simulink library "SLUGS_Library"  (Simulink 7.8)
settings: Solver=ode45  SolverMode=SingleTasking  StartTime=0.0  StopTime=10.0  RelTol=1e-3
values from neighbouring files (symbols this model uses):
  apSampleTime = 0.01    [mcuInit.m]
  derivativesConstant = 5    [mcuInit.m]
  latlong_WP = 1    [mcuInit.m]
  T = 0.01    [mcuInit.m]
  Xpoints = [0 0]    [mcuInit.m]
  Ypoints = [0 0]    [mcuInit.m]
  Zpoints = [0 0]    [mcuInit.m]
undefined symbols (not defined in the file or in its folder): bankCommandLimit, barAdjust, baroCutTemp, baroOffset, baroScale, barTGain1, barTGain2, barTMean1, barTMean2, baseHeight, baseTemp, daLimit, deLimit, DiscIntNeverNeededParam, drLimit, dtLimit, gaind, getGSLocation, getWP, GS_location, Init_onlyOnce, Init_Reset, IPStar, ISA_g, lapseRate, mass, maxAcc, MaxDwnPthStar, maxDynPressure, maxEta, Ndelay, param, pitAdjust, pitchCommandLimit, pitCutTemp, pitotOffset, pitotScale, pitTGain1, pitTGain2, pitTMean1, pitTMean2, polesd, pressureSensorCutoff, rollControlLimit, SampleT, setDiagnosticFloat, setDiagnosticShort, setLogFloat1, setLogFloat2, setNavLong, setNavNav, tanIntercept, Ts, u1, y1, yawDamperLimit, yo, zerosd
libraries: SLUGS_Library x90, simulink x37, dsPICdrivers x33, aerolibconvert2 x4, aerolibutil x1, aerolibobsolete x1
(part 1 of 7)
settings Model: Creator=Administrator  LastModifiedBy=User

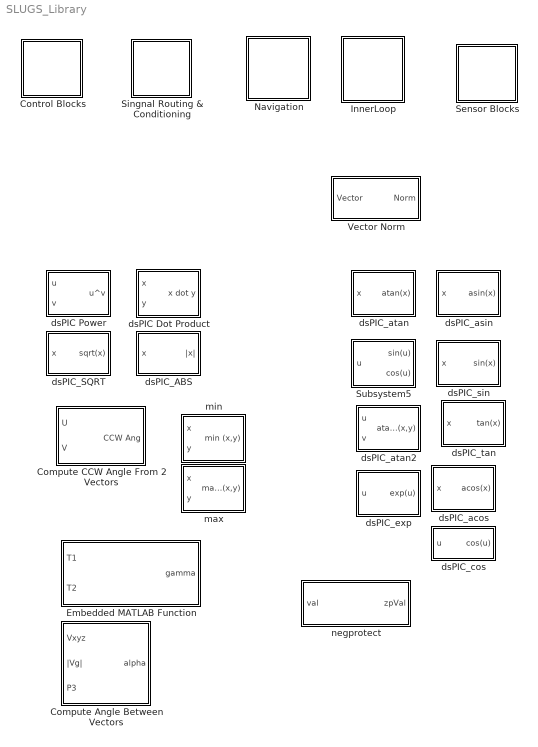
== system SLUGS_Library ==
  Compute Angle Between Vectors : Subsystem
  Compute CCW Angle From 2 Vectors : Subsystem
  Control Blocks : Subsystem
  Embedded MATLAB Function : MATLAB Function  TreatAsAtomicUnit=on
  InnerLoop : Subsystem
  Navigation : Subsystem
  Sensor Blocks : Subsystem  AncestorBlock=SLUGS_Library/Control Blocks
  Singnal Routing & Conditioning : Subsystem
  Subsystem5 : Subsystem
  Vector Norm : Subsystem
  dsPIC Dot Product : Subsystem
  dsPIC Power : Subsystem  AncestorBlock=SLUGS_Library/Air Density from Height/Subsystem
  dsPIC_ABS : Subsystem
  dsPIC_SQRT : Subsystem  AncestorBlock=SLUGS_Library/Compute Airspeed/Subsystem
  dsPIC_acos : Subsystem
  dsPIC_asin : Subsystem  AncestorBlock=SLUGS_Library/Subsystem2
  dsPIC_atan : Subsystem
  dsPIC_atan2 : Subsystem  AncestorBlock=SLUGS_Library/Air Density from Height/Subsystem
  dsPIC_cos : Subsystem  AncestorBlock=SLUGS_Library/Subsystem5
  dsPIC_exp : Subsystem  AncestorBlock=SLUGS_Library/Subsystem11
  dsPIC_sin : Subsystem  AncestorBlock=SLUGS_Library/Subsystem2
  dsPIC_tan : Subsystem
  max : Subsystem  AncestorBlock=SLUGS_Library/Subsystem3
  min : Subsystem  AncestorBlock=SLUGS_Library/Subsystem3
  negprotect : MATLAB Function  TreatAsAtomicUnit=on

== system SLUGS_Library/Compute Angle Between Vectors ==
  Vxyz : Inport
  |Vg| : Inport  Port=2
  P3 : Inport  Port=3
  Product8 : Product  Inputs=*/  RndMeth=Zero
  Product9 : Product  RndMeth=Zero
  Vector Norm : SLUGS_Library/Vector Norm
  "[-1 1]" : Saturate  UpperLimit=1  LowerLimit=-1
  dsPIC Dot Product : SLUGS_Library/dsPIC Dot Product
  dsPIC_acos : SLUGS_Library/dsPIC_acos
  negprotect3 : MATLAB Function  TreatAsAtomicUnit=on
  alpha : Outport
  wires:
  P3/1 -> dsPIC Dot Product/2, Vector Norm/1
  Vxyz/1 -> dsPIC Dot Product/1
  dsPIC Dot Product/1 -> Product8/1
  Vector Norm/1 -> Product9/1
  |Vg|/1 -> Product9/2
  Product9/1 -> negprotect3/1(val)
  Product8/1 -> "[-1 1]"/1
  "[-1 1]"/1 -> dsPIC_acos/1
  negprotect3/1(zpVal) -> Product8/2
  dsPIC_acos/1 -> alpha/1

== system SLUGS_Library/Compute CCW Angle From 2 Vectors ==
  U : Inport
  V : Inport  Port=2
  Add : Sum  Inputs=+-
  Embedded MATLAB Function1 : MATLAB Function  TreatAsAtomicUnit=on
  Selector : Selector  InputPortWidth=3  IndexOptions=Index vector (dialog)  Indices=[1]  OutputSizes=1
  Selector1 : Selector  InputPortWidth=3  IndexOptions=Index vector (dialog)  Indices=[1]  OutputSizes=1
  Selector2 : Selector  InputPortWidth=3  IndexOptions=Index vector (dialog)  Indices=[2]  OutputSizes=1
  Selector3 : Selector  InputPortWidth=3  IndexOptions=Index vector (dialog)  Indices=[2]  OutputSizes=1
  Subsystem1 : SLUGS_Library/Subsystem4
  Subsystem4 : SLUGS_Library/Subsystem4
  CCW Ang : Outport
  wires:
  Embedded MATLAB Function1/1(angle) -> CCW Ang/1
  V/1 -> Selector1/1, Selector2/1
  U/1 -> Selector/1, Selector3/1
  Add/1 -> Embedded MATLAB Function1/1(rawAngle)
  Subsystem1/1 -> Add/2
  Subsystem4/1 -> Add/1
  Selector1/1 -> Subsystem1/2
  Selector2/1 -> Subsystem1/1
  Selector/1 -> Subsystem4/2
  Selector3/1 -> Subsystem4/1

== system SLUGS_Library/Control Blocks ==
  Control Blocks Examples : Subsystem  AncestorBlock=SLUGS_Library/Control Blocks
  Lateral Channel : Subsystem
  Longitudinal Channel : Subsystem
  psi_dot_c Select logic : Subsystem

== system SLUGS_Library/InnerLoop ==
  Lateral Channel : Subsystem  TreatAsAtomicUnit=on
  Longitudinal Channel : Subsystem  TreatAsAtomicUnit=on
  Navigation : Subsystem  TreatAsAtomicUnit=on

== system SLUGS_Library/Navigation ==
  Bank to Psi Dot : Subsystem
  Compute Lateral Error : Subsystem
  Compute Distance : Subsystem  AncestorBlock=SLUGS_Library/Navigation/Compute Distance
  Compute Frenet : Subsystem
  Compute WP Index : Subsystem  AncestorBlock=SLUGS_Library/Navigation/Compute WP Index
  Dot Product : DotProduct  InputSameDT=on  OutDataTypeStr=Inherit: Inherit via internal rule
  Geod2LTP : Subsystem
      mask Description:
      | This block provides transformation of the Geodetic coordinates
      | to the LTP coorinate system. The block uses two consecutive transformations
      | (Geodetic -> ECEF ->LTP).
      | Geodetic coordinates of the LTP origin should also be predetermined.
      mask Help: Oops!
      mask Display: plot(0,0,100,100,[45,40,35,40,40],[85,95,85,95,40],[85,95,85,95,40],[35,40,45,40,40],[60,40,10,20,10,14],[70,40,10,13,10,20],[56,45],[70,70],[60,60],[50,60],[60,60],[30,40],[50,60],[20,20],[30,40],[20,20],[45,55],[35,25],[75,65],[35,25])
  Navigation : Subsystem
  Norm : Subsystem  AncestorBlock=SLUGS_Library/Navigation/Norm
  Normalize Vector : Subsystem
  "Park, Deyst & How Lat Accel Cmd" : Subsystem  AncestorBlock=SLUGS_Library/Navigation/Park, Deyst & How Lat Accel Cmd
  as_c to phi_c : Subsystem
  get WP Coord from Index : Subsystem
  psi_dot to Bank : Subsystem

== system SLUGS_Library/Sensor Blocks ==
  Baro Alt : Subsystem
  Pitot Control End : Subsystem
  Pitot Sensor End : Subsystem

== system SLUGS_Library/Singnal Routing & Conditioning ==
  3D Filter : Subsystem  RTWFcnName=TustinFilter3D  mask{zval=[], pval=-5, kval=5, TSample=0.01}
      mask prompts: zval "Zeros"; pval "Poles"; kval "Gains"; TSample "Sample Time"
      settings: RTWFcnNameOpts=User specified  RTWFileNameOpts=Use function name
      mask Display:
      | droots(zval,pval,kval)
      | port_label('input',1,'3D')
  3D LowPass w/Initial Condition : Subsystem  mask{a=5, yo=yo}
      mask prompts: a "Pole Location (continous)"; yo "Initial condition (3x1)"
      mask help: 3D Discrete 1st Order Low Pass filter
      mask Display:
      | port_label('input',1,'3D')
      | dpoly([a],[1 a],'s')
  Discrete Low Pass w/initial condition : Subsystem  mask{a=0.5, Yo=yo, Ts=T}
      mask prompts: a "Pole location (continuous)"; Yo "Initial condition"; Ts "Sample Time (seconds)"
      mask Display:
      | port_label('input',1,'U')
      | port_label('output',1,'Y')
      | text(0.35,0.85,'Tustin')
      | dpoly([a],[1 a],'s')
  Ellipse Correction : Subsystem  AncestorBlock=SLUGS_Library/Singnal Routing & Conditioning/Ellipse Correction  mask{param=param}
      mask prompts: param "parameter (struct)"
      mask help: Applies the correction from the ellipse algorithm to the raw data being sent through the block. The block expects a 3x1 input vector, and will return a 3x1 output vector. The parameter constant should be a struct with param.xo .yo and .zo being the offsets, param.a .b and .c being the scale factors, and param.phi .rho and .lambda being the angle non-orthogonality (in degrees).
      mask Display:
      | text(0.2,0.85,'Ellipse Correction')
      | port_label('input',1,'RAW')
      | port_label('output',1,'CORR')
  Filter : Subsystem  mask(DiscretizedZeroPole){Zeros=[], Poles=[-5], Gain=5, AbsTol=auto, SampleTime=SampleT, method=tustin, Wc=1}
      mask prompts: Zeros "Zeros (enter in s-main:)"; Poles "Poles (enter in s-domain:)"; Gain "Gain (enter in s-domain:)"; AbsTol "Absolute tolerance:"; SampleTime "Sample time:"; Wc "Critical Frequency (Hz):"
      mask help: Continuous mask uses c2d to transform parameters onto the Discrete Zero-Pole block inside.
      mask init:
      | st=SampleTime;
      | if length(st)>1
      |     st=SampleTime(1);
      | end
      | if(st>0)
      |     [zerosd,polesd,gaind] = sldiscutil('disczpk', {st,method,Wc,Zeros,Poles,Gain});
      | end	
      | s = get_param(gcb,'maskvalues');
      | zeross = s{1};
      | poless = s{2};
      | gainss = s{3};
      | %zerosc = eval(zeross);
      | %polesc = eval(poless);
      | %gainsc = eval(gainss);
      | sldiscutil('initzpkmask', st);
      | if(st==0)
      | set_param([gcb '/Zero Pole'], 'AbsoluteTolerance', AbsTol);
      | end
      mask StyleString: edit,edit,edit,edit,edit,popup(zoh|foh|tustin|prewarp|matched),edit
      mask CallbackString: |||||hidecrit|
      mask Display:
      | droots(zeross,poless,gainss)
      | text( 0.5, 1.0, method, 'verticalAlignment','top')
  Rate Limiter Dynamic with External IC : Subsystem  mask{rlIC=0}
  Saturation : Saturate  SampleTime=SampleT
  Zero Limit : Subsystem
  myMux Fun3 : MATLAB Function  TreatAsAtomicUnit=on

== system SLUGS_Library/Subsystem5 ==
  u : Inport
  C Function Call : dsPICdrivers/OTHERS/C Function Call  Tag=dsPIC_dsPIC_CFunctionCall  FctUpdate=Output Function  fctName='mySin'  INPUT_SIZE=1  INPUT1=real32  INPUT2=--  INPUT3=--  OUTPUT_SIZE=1  OUTPUT1=real32  SampleTime=-1  InputType=[ 7 ]  OutputType=[ 7 ]  FctDeclaration=extern real32_T mySin(real32_T u1);  FctCall=%y1 = mySin(%u1);  OrderingInOutPopup=None  FctStart=None  FctStart_Name=Init_onlyOnce  FctStart_Declaration=inline extern void Init_onlyOnce();  FctStart_Call=Init_onlyOnce();  FctInit=None  FctInit_Name=Init_Reset  FctInit_Declaration=inline extern void Init_Reset();  FctInit_Call=Init_Reset();  PinDigitalInput=[]  PinDigitalOutput=[]  AnalogueInput=[]
  C Function Call1 : dsPICdrivers/OTHERS/C Function Call  Tag=dsPIC_dsPIC_CFunctionCall  FctUpdate=Output Function  fctName='myCos'  INPUT_SIZE=1  INPUT1=real32  INPUT2=--  INPUT3=--  OUTPUT_SIZE=1  OUTPUT1=real32  SampleTime=-1  InputType=[ 7 ]  OutputType=[ 7 ]  FctDeclaration=extern real32_T myCos(real32_T u1);  FctCall=%y1 = myCos(%u1);  OrderingInOutPopup=None  FctStart=None  FctStart_Name=Init_onlyOnce  FctStart_Declaration=inline extern void Init_onlyOnce();  FctStart_Call=Init_onlyOnce();  FctInit=None  FctInit_Name=Init_Reset  FctInit_Declaration=inline extern void Init_Reset();  FctInit_Call=Init_Reset();  PinDigitalInput=[]  PinDigitalOutput=[]  AnalogueInput=[]
  Environment Controller : simulink/Signal Routing/Environment Controller
  Environment Controller1 : simulink/Signal Routing/Environment Controller
  SinCos1 : aerolibobsolete/SinCos
  sin(u) : Outport
  cos(u) : Outport  Port=2
  wires:
  SinCos1/2 -> Environment Controller1/1
  C Function Call1/1 -> Environment Controller1/2
  Environment Controller1/1 -> cos(u)/1
  u/1 -> C Function Call1/1, C Function Call/1, SinCos1/1
  SinCos1/1 -> Environment Controller/1
  C Function Call/1 -> Environment Controller/2
  Environment Controller/1 -> sin(u)/1

== system SLUGS_Library/Vector Norm ==
  Vector : Inport
  dsPIC Dot Product : SLUGS_Library/dsPIC Dot Product
  dsPIC_SQRT : SLUGS_Library/dsPIC_SQRT
  Norm : Outport
  wires:
  dsPIC Dot Product/1 -> dsPIC_SQRT/1
  Vector/1 -> dsPIC Dot Product/1, dsPIC Dot Product/2
  dsPIC_SQRT/1 -> Norm/1

== system SLUGS_Library/dsPIC Dot Product ==
  x : Inport
  y : Inport  Port=2
  Dot Product : DotProduct  InputSameDT=on  OutDataTypeStr=Inherit: Inherit via internal rule
  Embedded MATLAB Function : MATLAB Function  TreatAsAtomicUnit=on
  Environment Controller : simulink/Signal Routing/Environment Controller
  x dot y : Outport
  wires:
  y/1 -> Embedded MATLAB Function/2(y), Dot Product/2
  x/1 -> Embedded MATLAB Function/1(x), Dot Product/1
  Dot Product/1 -> Environment Controller/1
  Embedded MATLAB Function/1(xDoty) -> Environment Controller/2
  Environment Controller/1 -> x dot y/1

== system SLUGS_Library/dsPIC Power ==
  u : Inport
  v : Inport  Port=2
  C Function Call : dsPICdrivers/OTHERS/C Function Call  Tag=dsPIC_dsPIC_CFunctionCall  FctUpdate=Output Function  fctName='myPow'  INPUT_SIZE=1  INPUT1=real32  INPUT2=real32  INPUT3=--  OUTPUT_SIZE=1  OUTPUT1=real32  SampleTime=-1  InputType=[ 7 7 ]  OutputType=[ 7 ]  FctDeclaration=extern real32_T myPow(real32_T u1, real32_T u2);  FctCall=%y1 = myPow(%u1, %u2);  OrderingInOutPopup=None  FctStart=None  FctStart_Name=Init_onlyOnce  FctStart_Declaration=inline extern void Init_onlyOnce();  FctStart_Call=Init_onlyOnce();  FctInit=None  FctInit_Name=Init_Reset  FctInit_Declaration=inline extern void Init_Reset();  FctInit_Call=Init_Reset();  PinDigitalInput=[]  PinDigitalOutput=[]  AnalogueInput=[]
  Environment Controller : simulink/Signal Routing/Environment Controller
  Math Function : Math  Operator=pow  SaturateOnIntegerOverflow=on
  u^v : Outport
  wires:
  u/1 -> C Function Call/1, Math Function/1
  v/1 -> C Function Call/2, Math Function/2
  Math Function/1 -> Environment Controller/1
  C Function Call/1 -> Environment Controller/2
  Environment Controller/1 -> u^v/1

== system SLUGS_Library/dsPIC_ABS ==
  x : Inport
  Abs : Abs
  C Function Call : dsPICdrivers/OTHERS/C Function Call  Tag=dsPIC_dsPIC_CFunctionCall  FctUpdate=Output Function  fctName='myAbs'  INPUT_SIZE=1  INPUT1=real32  INPUT2=--  INPUT3=--  OUTPUT_SIZE=1  OUTPUT1=real32  SampleTime=-1  InputType=[ 7 ]  OutputType=[ 7 ]  FctDeclaration=extern real32_T myAbs(real32_T u1);  FctCall=%y1 = myAbs(%u1);  OrderingInOutPopup=None  FctStart=None  FctStart_Name=Init_onlyOnce  FctStart_Declaration=inline extern void Init_onlyOnce();  FctStart_Call=Init_onlyOnce();  FctInit=None  FctInit_Name=Init_Reset  FctInit_Declaration=inline extern void Init_Reset();  FctInit_Call=Init_Reset();  PinDigitalInput=[]  PinDigitalOutput=[]  AnalogueInput=[]
  Environment Controller : simulink/Signal Routing/Environment Controller
  |x| : Outport
  wires:
  x/1 -> Abs/1, C Function Call/1
  C Function Call/1 -> Environment Controller/2
  Abs/1 -> Environment Controller/1
  Environment Controller/1 -> |x|/1

== system SLUGS_Library/dsPIC_SQRT ==
  x : Inport
  C Function Call : dsPICdrivers/OTHERS/C Function Call  Tag=dsPIC_dsPIC_CFunctionCall  FctUpdate=Output Function  fctName='mySqrt'  INPUT_SIZE=1  INPUT1=real32  INPUT2=--  INPUT3=--  OUTPUT_SIZE=1  OUTPUT1=real32  SampleTime=-1  InputType=[ 7 ]  OutputType=[ 7 ]  FctDeclaration=extern real32_T mySqrt(real32_T u1);  FctCall=%y1 = mySqrt(%u1);  OrderingInOutPopup=None  FctStart=None  FctStart_Name=Init_onlyOnce  FctStart_Declaration=inline extern void Init_onlyOnce();  FctStart_Call=Init_onlyOnce();  FctInit=None  FctInit_Name=Init_Reset  FctInit_Declaration=inline extern void Init_Reset();  FctInit_Call=Init_Reset();  PinDigitalInput=[]  PinDigitalOutput=[]  AnalogueInput=[]
  Environment Controller : simulink/Signal Routing/Environment Controller
  Math Function1 : Math  Operator=sqrt  SaturateOnIntegerOverflow=on
  negprotect : MATLAB Function  TreatAsAtomicUnit=on
  sqrt(x) : Outport
  wires:
  C Function Call/1 -> Environment Controller/2
  Math Function1/1 -> Environment Controller/1
  Environment Controller/1 -> sqrt(x)/1
  negprotect/1(zpVal) -> C Function Call/1, Math Function1/1
  x/1 -> negprotect/1(val)

== system SLUGS_Library/dsPIC_acos ==
  x : Inport
  C Function Call : dsPICdrivers/OTHERS/C Function Call  Tag=dsPIC_dsPIC_CFunctionCall  FctUpdate=Output Function  fctName='myAcos'  INPUT_SIZE=1  INPUT1=real32  INPUT2=--  INPUT3=--  OUTPUT_SIZE=1  OUTPUT1=real32  SampleTime=-1  InputType=[ 7 ]  OutputType=[ 7 ]  FctDeclaration=extern real32_T myAcos(real32_T u1);  FctCall=%y1 = myAcos(%u1);  OrderingInOutPopup=None  FctStart=None  FctStart_Name=Init_onlyOnce  FctStart_Declaration=inline extern void Init_onlyOnce();  FctStart_Call=Init_onlyOnce();  FctInit=None  FctInit_Name=Init_Reset  FctInit_Declaration=inline extern void Init_Reset();  FctInit_Call=Init_Reset();  PinDigitalInput=[]  PinDigitalOutput=[]  AnalogueInput=[]
  Environment Controller : simulink/Signal Routing/Environment Controller
  Trigonometric Function : Trigonometry  Operator=acos
  acos(x) : Outport
  wires:
  x/1 -> C Function Call/1, Trigonometric Function/1
  Trigonometric Function/1 -> Environment Controller/1
  C Function Call/1 -> Environment Controller/2
  Environment Controller/1 -> acos(x)/1

== system SLUGS_Library/dsPIC_asin ==
  x : Inport
  C Function Call : dsPICdrivers/OTHERS/C Function Call  Tag=dsPIC_dsPIC_CFunctionCall  FctUpdate=Output Function  fctName='myAsin'  INPUT_SIZE=1  INPUT1=real32  INPUT2=--  INPUT3=--  OUTPUT_SIZE=1  OUTPUT1=real32  SampleTime=-1  InputType=[ 7 ]  OutputType=[ 7 ]  FctDeclaration=extern real32_T myAsin(real32_T u1);  FctCall=%y1 = myAsin(%u1);  OrderingInOutPopup=None  FctStart=None  FctStart_Name=Init_onlyOnce  FctStart_Declaration=inline extern void Init_onlyOnce();  FctStart_Call=Init_onlyOnce();  FctInit=None  FctInit_Name=Init_Reset  FctInit_Declaration=inline extern void Init_Reset();  FctInit_Call=Init_Reset();  PinDigitalInput=[]  PinDigitalOutput=[]  AnalogueInput=[]
  Environment Controller : simulink/Signal Routing/Environment Controller
  Trigonometric Function : Trigonometry  Operator=asin
  "[-1,1]" : Saturate  UpperLimit=0.9999  LowerLimit=-0.999
  asin(x) : Outport
  wires:
  Environment Controller/1 -> asin(x)/1
  C Function Call/1 -> Environment Controller/2
  Trigonometric Function/1 -> Environment Controller/1
  x/1 -> "[-1,1]"/1
  "[-1,1]"/1 -> Trigonometric Function/1, C Function Call/1

== system SLUGS_Library/dsPIC_atan ==
  x : Inport
  C Function Call : dsPICdrivers/OTHERS/C Function Call  Tag=dsPIC_dsPIC_CFunctionCall  FctUpdate=Output Function  fctName='myAtan'  INPUT_SIZE=1  INPUT1=real32  INPUT2=--  INPUT3=--  OUTPUT_SIZE=1  OUTPUT1=real32  SampleTime=-1  InputType=[ 7 ]  OutputType=[ 7 ]  FctDeclaration=extern real32_T myAtan(real32_T u1);  FctCall=%y1 = myAtan(%u1);  OrderingInOutPopup=None  FctStart=None  FctStart_Name=Init_onlyOnce  FctStart_Declaration=inline extern void Init_onlyOnce();  FctStart_Call=Init_onlyOnce();  FctInit=None  FctInit_Name=Init_Reset  FctInit_Declaration=inline extern void Init_Reset();  FctInit_Call=Init_Reset();  PinDigitalInput=[]  PinDigitalOutput=[]  AnalogueInput=[]
  Environment Controller : simulink/Signal Routing/Environment Controller
  Trigonometric Function : Trigonometry  Operator=atan
  atan(x) : Outport
  wires:
  Environment Controller/1 -> atan(x)/1
  C Function Call/1 -> Environment Controller/2
  Trigonometric Function/1 -> Environment Controller/1
  x/1 -> Trigonometric Function/1, C Function Call/1

== system SLUGS_Library/dsPIC_atan2 ==
  u : Inport
  v : Inport  Port=2
  C Function Call : dsPICdrivers/OTHERS/C Function Call  Tag=dsPIC_dsPIC_CFunctionCall  FctUpdate=Output Function  fctName='myAtan2'  INPUT_SIZE=1  INPUT1=real32  INPUT2=real32  INPUT3=--  OUTPUT_SIZE=1  OUTPUT1=real32  SampleTime=-1  InputType=[ 7 7 ]  OutputType=[ 7 ]  FctDeclaration=extern real32_T myAtan2(real32_T u1, real32_T u2);  FctCall=%y1 = myAtan2(%u1, %u2);  OrderingInOutPopup=None  FctStart=None  FctStart_Name=Init_onlyOnce  FctStart_Declaration=inline extern void Init_onlyOnce();  FctStart_Call=Init_onlyOnce();  FctInit=None  FctInit_Name=Init_Reset  FctInit_Declaration=inline extern void Init_Reset();  FctInit_Call=Init_Reset();  PinDigitalInput=[]  PinDigitalOutput=[]  AnalogueInput=[]
  Environment Controller : simulink/Signal Routing/Environment Controller
  Trigonometric Function : Trigonometry  Operator=atan2
  atan2(x,y) : Outport
  wires:
  u/1 -> Trigonometric Function/1, C Function Call/1
  v/1 -> Trigonometric Function/2, C Function Call/2
  Trigonometric Function/1 -> Environment Controller/1
  C Function Call/1 -> Environment Controller/2
  Environment Controller/1 -> atan2(x,y)/1

== system SLUGS_Library/dsPIC_cos ==
  u : Inport
  Environment Controller1 : simulink/Signal Routing/Environment Controller
  Trigonometric Function : Trigonometry  Operator=cos
  "[apUtils.c]" : dsPICdrivers/OTHERS/C Function Call  Tag=dsPIC_dsPIC_CFunctionCall  FctUpdate=Output Function  fctName='myCos'  INPUT_SIZE=1  INPUT1=real32  INPUT2=--  INPUT3=--  OUTPUT_SIZE=1  OUTPUT1=real32  SampleTime=-1  InputType=[ 7 ]  OutputType=[ 7 ]  FctDeclaration=extern real32_T myCos(real32_T u1);  FctCall=%y1 = myCos(%u1);  OrderingInOutPopup=None  FctStart=None  FctStart_Name=Init_onlyOnce  FctStart_Declaration=inline extern void Init_onlyOnce();  FctStart_Call=Init_onlyOnce();  FctInit=None  FctInit_Name=Init_Reset  FctInit_Declaration=inline extern void Init_Reset();  FctInit_Call=Init_Reset();  PinDigitalInput=[]  PinDigitalOutput=[]  AnalogueInput=[]
  cos(u) : Outport
  wires:
  Trigonometric Function/1 -> Environment Controller1/1
  "[apUtils.c]"/1 -> Environment Controller1/2
  Environment Controller1/1 -> cos(u)/1
  u/1 -> Trigonometric Function/1, "[apUtils.c]"/1

== system SLUGS_Library/dsPIC_exp ==
  u : Inport
  C Function Call : dsPICdrivers/OTHERS/C Function Call  Tag=dsPIC_dsPIC_CFunctionCall  FctUpdate=Output Function  fctName='myExp'  INPUT_SIZE=1  INPUT1=real32  INPUT2=--  INPUT3=--  OUTPUT_SIZE=1  OUTPUT1=real32  SampleTime=-1  InputType=[ 7 ]  OutputType=[ 7 ]  FctDeclaration=extern real32_T myExp(real32_T u1);  FctCall=%y1 = myExp(%u1);  OrderingInOutPopup=None  FctStart=None  FctStart_Name=Init_onlyOnce  FctStart_Declaration=inline extern void Init_onlyOnce();  FctStart_Call=Init_onlyOnce();  FctInit=None  FctInit_Name=Init_Reset  FctInit_Declaration=inline extern void Init_Reset();  FctInit_Call=Init_Reset();  PinDigitalInput=[]  PinDigitalOutput=[]  AnalogueInput=[]
  Environment Controller : simulink/Signal Routing/Environment Controller
  Math Function : Math  SaturateOnIntegerOverflow=on
  exp(u) : Outport
  wires:
  C Function Call/1 -> Environment Controller/2
  Environment Controller/1 -> exp(u)/1
  u/1 -> C Function Call/1, Math Function/1
  Math Function/1 -> Environment Controller/1

== system SLUGS_Library/dsPIC_sin ==
  x : Inport
  C Function Call : dsPICdrivers/OTHERS/C Function Call  Tag=dsPIC_dsPIC_CFunctionCall  FctUpdate=Output Function  fctName='mySin'  INPUT_SIZE=1  INPUT1=real32  INPUT2=--  INPUT3=--  OUTPUT_SIZE=1  OUTPUT1=real32  SampleTime=-1  InputType=[ 7 ]  OutputType=[ 7 ]  FctDeclaration=extern real32_T mySin(real32_T u1);  FctCall=%y1 = mySin(%u1);  OrderingInOutPopup=None  FctStart=None  FctStart_Name=Init_onlyOnce  FctStart_Declaration=inline extern void Init_onlyOnce();  FctStart_Call=Init_onlyOnce();  FctInit=None  FctInit_Name=Init_Reset  FctInit_Declaration=inline extern void Init_Reset();  FctInit_Call=Init_Reset();  PinDigitalInput=[]  PinDigitalOutput=[]  AnalogueInput=[]
  Environment Controller : simulink/Signal Routing/Environment Controller
  Trigonometric Function : Trigonometry
  sin(x) : Outport
  wires:
  Environment Controller/1 -> sin(x)/1
  C Function Call/1 -> Environment Controller/2
  Trigonometric Function/1 -> Environment Controller/1
  x/1 -> Trigonometric Function/1, C Function Call/1

== system SLUGS_Library/dsPIC_tan ==
  x : Inport
  C Function Call : dsPICdrivers/OTHERS/C Function Call  Tag=dsPIC_dsPIC_CFunctionCall  FctUpdate=Output Function  fctName='myTan'  INPUT_SIZE=1  INPUT1=real32  INPUT2=--  INPUT3=--  OUTPUT_SIZE=1  OUTPUT1=real32  SampleTime=-1  InputType=[ 7 ]  OutputType=[ 7 ]  FctDeclaration=extern real32_T myTan(real32_T u1);  FctCall=%y1 = myTan(%u1);  OrderingInOutPopup=None  FctStart=None  FctStart_Name=Init_onlyOnce  FctStart_Declaration=inline extern void Init_onlyOnce();  FctStart_Call=Init_onlyOnce();  FctInit=None  FctInit_Name=Init_Reset  FctInit_Declaration=inline extern void Init_Reset();  FctInit_Call=Init_Reset();  PinDigitalInput=[]  PinDigitalOutput=[]  AnalogueInput=[]
  Environment Controller : simulink/Signal Routing/Environment Controller
  Trigonometric Function : Trigonometry  Operator=tan
  tan(x) : Outport
  wires:
  x/1 -> C Function Call/1, Trigonometric Function/1
  Trigonometric Function/1 -> Environment Controller/1
  C Function Call/1 -> Environment Controller/2
  Environment Controller/1 -> tan(x)/1

== system SLUGS_Library/max ==
  x : Inport
  y : Inport  Port=2
  Relational Operator : RelationalOperator  Operator=>  OutDataTypeStr=boolean
  Switch : Switch  Threshold=0.5
  max (x,y) : Outport
  wires:
  x/1 -> Relational Operator/1, Switch/1
  y/1 -> Relational Operator/2, Switch/3
  Relational Operator/1 -> Switch/2
  Switch/1 -> max (x,y)/1

== system SLUGS_Library/min ==
  x : Inport
  y : Inport  Port=2
  Relational Operator : RelationalOperator  Operator=<  OutDataTypeStr=boolean
  Switch : Switch  Threshold=0.5
  min (x,y) : Outport
  wires:
  Switch/1 -> min (x,y)/1
  Relational Operator/1 -> Switch/2
  y/1 -> Switch/3, Relational Operator/2
  x/1 -> Switch/1, Relational Operator/1

== system SLUGS_Library/Control Blocks/Control Blocks Examples ==
  PD Controller  Internal Derivative : Subsystem  mask{TSample=SampleT, NDelay=5}
      mask prompts: TSample "Sample Time"; NDelay "Derivation Time Constant Factor (1->10)"
      mask help:
      | This Block implements a PD Controller with the Following Characteristcs:
      |
      | 1.- It still expects 3 values for Gains. The second term (I) is ignored
      | 2.- The time Derivative is "low-passed" by using the previous N samples instead of the one before
  PD Controller  no Internal Derivative : Subsystem  mask{TSample=SampleT}
      mask prompts: TSample "Sample Time"
      mask help:
      | This Block implements a PD Controller with the Following Characteristcs:
      |
      | 1.- It still expects 3 values for Gains. The second term (I) is ignored
      | 2.- The time Derivative is "low-passed" by using the previous N samples instead of the one before
  PI Controller : Subsystem  mask{TSample=SampleT, upperLimit=10, lowerLimit=-10}
      mask prompts: TSample "Sample Time"; upperLimit "Integrator Upper Windup Limit"; lowerLimit "Integrator Lower Windup Limit"
      mask help:
      | This Block implements a PI Controller with the Following Characteristcs:
      |
      | 1.- Integrator antiwindup is given by the limits in the block
      | 2.-The gain still expects 3 values (the D term is ignored)
      | 3.- It contains an Integrator Reset if needed
  PI Controller w/Anti-Windup : Subsystem  mask(PID){Tsample=Ts, Ndelay=Ndelay, upperSaturationLimit=deLimit, lowerSaturationLimit=0}
      mask prompts: Tsample "Sample Time"; Ndelay "Integer delays for de/dt"; upperSaturationLimit "Upper Saturation Limit"; lowerSaturationLimit "Lower Saturation Limit"
      mask help: PID controller block with anti-windup and saturation limits. Implemented as a discrete forwardl integration which stops integrating when the output is saturated. Derivative is implemented as a numerical derivative with N integer delays to smooth output.
      mask Display:
      | disp('PI')
      | port_label('input',1,'error')
      | port_label('input',3,'gains')
      | port_label('input',2,'reset')
      | port_label('input',4,'trim')
      | port_label('output',1,'output')
  PID Controller : Subsystem  mask{TSample=SampleT, NDelay=5, upperLimit=10, lowerLimit=-10}
      mask prompts: TSample "Sample Time"; NDelay "Derivation Time Constant Factor (1->10)"; upperLimit "Integrator Upper Windup Limit"; lowerLimit "Integrator Lower Windup Limit"
      mask help:
      | This Block implements a PID Controller with the Following Characteristcs:
      |
      | 1.- Integrator antiwindup is given by the limits in the block
      | 2.- The time Derivative is "low-passed" by using the previous N samples instead of the one before
      | 3.- It contains an Integrator Reset if needed
  PID Controller no Internal Derivative : Subsystem  mask{TSample=SampleT, upperLimit=10, lowerLimit=-10}
      mask prompts: TSample "Sample Time"; upperLimit "Integrator Upper Windup Limit"; lowerLimit "Integrator Lower Windup Limit"
      mask help:
      | This Block implements a PID Controller with the Following Characteristcs:
      |
      | 1.- Integrator antiwindup is given by the limits in the block
      | 2.- The error time derivative is provided and therefore no derivtive block is implemented
      | 3.- It contains an Integrator Reset if needed
  PID Controller w/Anti-Windup : Subsystem  mask(PID){Tsample=Ts, Ndelay=Ndelay, upperSaturationLimit=deLimit, lowerSaturationLimit=0}
      mask prompts: Tsample "Sample Time"; Ndelay "Integer delays for de/dt"; upperSaturationLimit "Upper Saturation Limit"; lowerSaturationLimit "Lower Saturation Limit"
      mask help: PID controller block with anti-windup and saturation limits. Implemented as a discrete forwardl integration which stops integrating when the output is saturated. Derivative is implemented as a numerical derivative with N integer delays to smooth output.
      mask Display:
      | disp('PID')
      | port_label('input',1,'error')
      | port_label('input',3,'gains')
      | port_label('input',2,'reset')
      | port_label('input',4,'trim')
      | port_label('output',1,'output')
  PID available Derivative w/Anti-Windup : Subsystem  mask(PID){Tsample=Ts, Ndelay=Ndelay, SaturationLimit=deLimit}
      mask prompts: Tsample "Sample Time"; Ndelay "Integer delays for de/dt"; SaturationLimit "Saturation Limit"
      mask help: PID controller block with anti-windup and saturation limits. Implemented as a discrete forwardl integration which stops integrating when the output is saturated. Derivative is implemented as a numerical derivative with N integer delays to smooth output.
      mask Display:
      | disp('PID')
      | port_label('input',1,'error')
      | port_label('input',2,'de/dt')
      | port_label('input',3,'gains')
      | port_label('input',4,'reset')
      | port_label('output',1,'output')

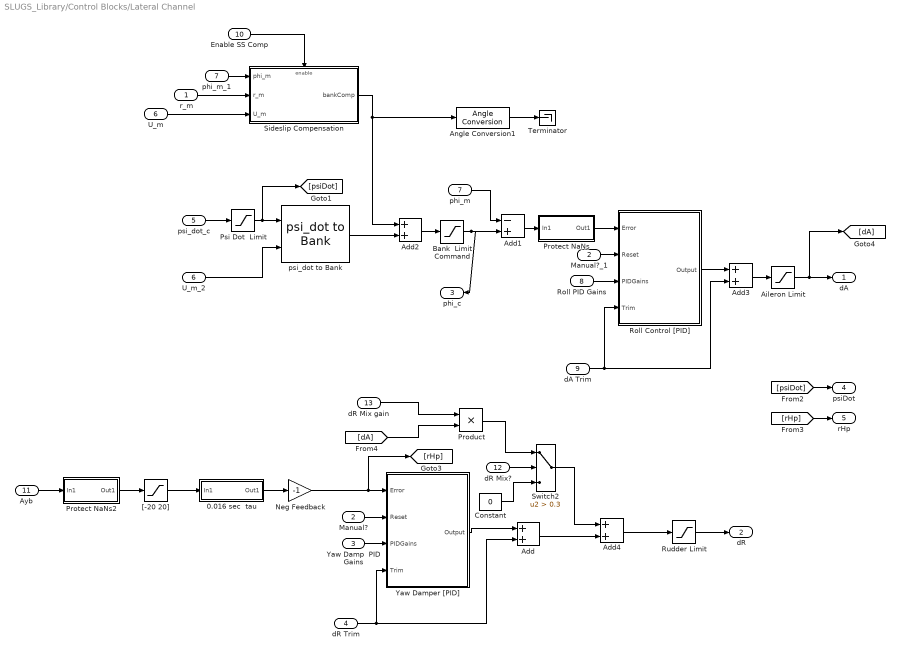
== system SLUGS_Library/Control Blocks/Lateral Channel ==
  r_m : Inport
  Manual? : Inport  Port=2
  Yaw Damp  PID Gains : Inport  Port=3
  dR Trim : Inport  Port=4
  psi_dot_c : Inport  Port=5
  U_m : Inport  Port=6
  phi_m : Inport  Port=7
  Roll PID Gains : Inport  Port=8
  dA Trim : Inport  Port=9
  Enable SS Comp : Inport  Port=10
  Ayb : Inport  Port=11
  dR Mix? : Inport  Port=12
  dR Mix gain : Inport  Port=13
  0.016 sec  tau : Subsystem  mask(Tustin1stOrderLowpassAutoInitialCondition){f=10, T=T}
      mask prompts: f "Lowpass Frequency"; T "Sample Time"
      mask help: Takes a 3db rolloff frequency (in Hz, NOT radians/s) and a sample time. Performs a symbolic Tustin conversion and implements in a discrete filter. The initial output of the filter is set by the first sample.
      mask Help: Enter the desired 3db rolloff frequency in Hz and the sample time. Initial conditions are sampled automatically.
      mask Display: fprintf('%.2f Hz lowpass',f)
  Add{,2..4} (4 alike) : Sum  OutDataTypeStr=single
  Add1 : Sum  Inputs=-+  OutDataTypeStr=single
  Aileron Limit : Saturate  UpperLimit=daLimit  LowerLimit=-daLimit  SampleTime=apSampleTime
  Angle Conversion1 : aerolibconvert2/Angle Conversion  IU=rad  OU=deg
  Bank  Limit Command : Saturate  UpperLimit=bankCommandLimit  LowerLimit=-bankCommandLimit  SampleTime=apSampleTime
  Constant : Constant  Value=0  OutDataTypeStr=single
  Manual?_1 : InportShadow  Port=2
  "Neg Feedback " : Gain  Gain=-1  OutDataTypeStr=float('single')
  Product : Product  RndMeth=Zero
  Protect NaNs : Subsystem
  Protect NaNs2 : Subsystem
  Psi Dot  Limit : Saturate  UpperLimit=1  LowerLimit=-1  SampleTime=apSampleTime
  Roll Control [PID] : Subsystem  AncestorBlock=SLUGS_Library/Control Blocks/PID Controller w//Anti-Windup  mask(PID){Tsample=apSampleTime, Ndelay=derivativesConstant, upperSaturationLimit=daLimit, lowerSaturationLimit=-daLimit}
      mask prompts: Tsample "Sample Time"; Ndelay "Integer delays for de/dt"; upperSaturationLimit "Upper Saturation Limit"; lowerSaturationLimit "Lower Saturation Limit"
      mask help: PID controller block with anti-windup and saturation limits. Implemented as a discrete forwardl integration which stops integrating when the output is saturated. Derivative is implemented as a numerical derivative with N integer delays to smooth output.
      mask Display:
      | disp('PID')
      | port_label('input',1,'error')
      | port_label('input',3,'gains')
      | port_label('input',2,'reset')
      | port_label('input',4,'trim')
      | port_label('output',1,'output')
  Rudder Limit : Saturate  UpperLimit=drLimit  LowerLimit=-drLimit  SampleTime=apSampleTime
  Sideslip Compensation : Subsystem
  Switch2 : Switch  Criteria=u2 > Threshold  Threshold=0.3  InputSameDT=on
  Terminator : Terminator
  U_m_2 : InportShadow  Port=6
  Yaw Damper [PID] : Subsystem  AncestorBlock=SLUGS_Library/Control Blocks/PID Controller w//Anti-Windup  mask(PID){Tsample=apSampleTime, Ndelay=derivativesConstant, upperSaturationLimit=drLimit, lowerSaturationLimit=-drLimit}
      mask prompts: Tsample "Sample Time"; Ndelay "Integer delays for de/dt"; upperSaturationLimit "Upper Saturation Limit"; lowerSaturationLimit "Lower Saturation Limit"
      mask help: PID controller block with anti-windup and saturation limits. Implemented as a discrete forwardl integration which stops integrating when the output is saturated. Derivative is implemented as a numerical derivative with N integer delays to smooth output.
      mask Display:
      | disp('PID')
      | port_label('input',1,'error')
      | port_label('input',3,'gains')
      | port_label('input',2,'reset')
      | port_label('input',4,'trim')
      | port_label('output',1,'output')
  "[-20 20]" : Saturate  UpperLimit=20  LowerLimit=-20
  phi_m_1 : InportShadow  Port=7
  psi_dot to Bank : SLUGS_Library/Navigation/psi_dot to Bank
  dA : Outport
  dR : Outport  Port=2
  phi_c : Outport  Port=3
  psiDot : Outport  Port=4
  rHp : Outport  Port=5
  wires:
  psi_dot_c/1 -> Psi Dot  Limit/1
  Psi Dot  Limit/1 -> psi_dot to Bank/1, [psiDot]
  Bank  Limit Command/1 -> Add1/2, phi_c/1
  phi_m/1 -> Add1/1
  Add1/1 -> Protect NaNs/1(In1)
  Aileron Limit/1 -> dA/1, [dA]
  dA Trim/1 -> Add3/2, Roll Control [PID]/4(Trim)
  Roll Control [PID]/1(Output) -> Add3/1
  Add3/1 -> Aileron Limit/1
  Roll PID Gains/1 -> Roll Control [PID]/3(PIDGains)
  Manual?_1/1 -> Roll Control [PID]/2(Reset)
  dR Trim/1 -> Add/2, Yaw Damper [PID]/4(Trim)
  Yaw Damper [PID]/1(Output) -> Add/1
  Yaw Damp  PID Gains/1 -> Yaw Damper [PID]/3(PIDGains)
  Manual?/1 -> Yaw Damper [PID]/2(Reset)
  U_m_2/1 -> psi_dot to Bank/2
  Add2/1 -> Bank  Limit Command/1
  psi_dot to Bank/1 -> Add2/2
  Sideslip Compensation/1(bankComp) -> Add2/1, Angle Conversion1/1
  phi_m_1/1 -> Sideslip Compensation/1(phi_m)
  r_m/1 -> Sideslip Compensation/2(r_m)
  U_m/1 -> Sideslip Compensation/3(U_m)
  Enable SS Comp/1 -> Sideslip Compensation/Enable
  Ayb/1 -> Protect NaNs2/1(In1)
  "Neg Feedback "/1 -> [rHp], Yaw Damper [PID]/1(Error)
  0.016 sec  tau/1(Out1) -> "Neg Feedback "/1
  Rudder Limit/1 -> dR/1
  Protect NaNs/1(Out1) -> Roll Control [PID]/1(Error)
  Protect NaNs2/1(Out1) -> "[-20 20]"/1
  "[-20 20]"/1 -> 0.016 sec  tau/1(In1)
  Angle Conversion1/1 -> Terminator/1
  Add4/1 -> Rudder Limit/1
  Add/1 -> Add4/2
  Switch2/1 -> Add4/1
  dR Mix?/1 -> Switch2/2
  Constant/1 -> Switch2/3
  Product/1 -> Switch2/1
  dR Mix gain/1 -> Product/1
  [dA] -> Product/2
  [psiDot] -> psiDot/1
  [rHp] -> rHp/1

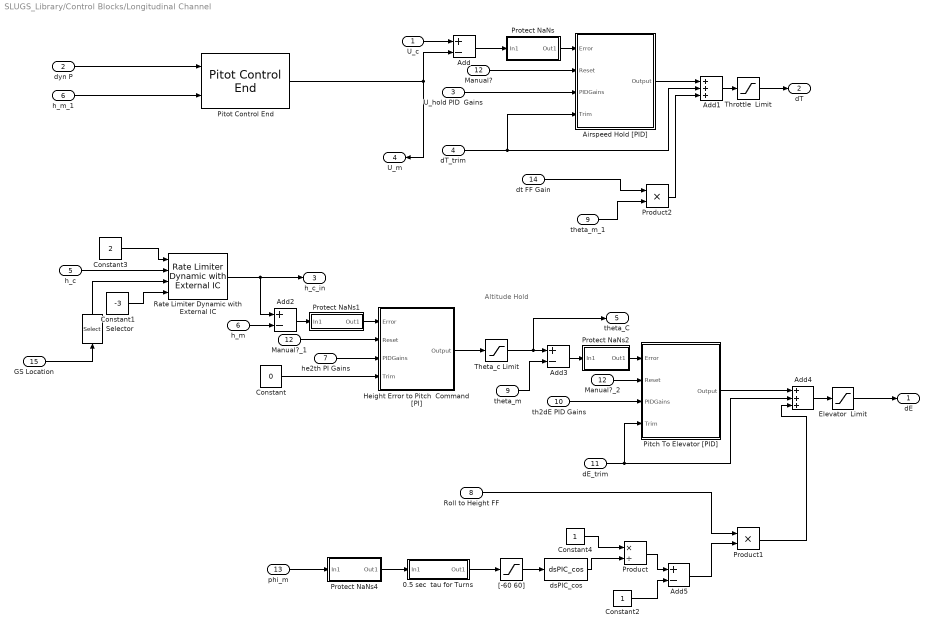
== system SLUGS_Library/Control Blocks/Longitudinal Channel ==
  note: Altitude Hold
  U_c : Inport
  dyn P : Inport  Port=2
  U_hold PID  Gains : Inport  Port=3
  dT_trim : Inport  Port=4
  h_c : Inport  Port=5
  h_m : Inport  Port=6
  he2th PI Gains : Inport  Port=7
  Roll to Height FF : Inport  Port=8
  theta_m : Inport  Port=9
  th2dE PID Gains : Inport  Port=10
  dE_trim : Inport  Port=11
  Manual? : Inport  Port=12
  phi_m : Inport  Port=13
  dt FF Gain : Inport  Port=14
  GS Location : Inport  Port=15
  0.5 sec  tau for Turns : Subsystem  mask(Tustin1stOrderLowpassAutoInitialCondition){f=0.32, T=T}
      mask prompts: f "Lowpass Frequency"; T "Sample Time"
      mask help: Takes a 3db rolloff frequency (in Hz, NOT radians/s) and a sample time. Performs a symbolic Tustin conversion and implements in a discrete filter. The initial output of the filter is set by the first sample.
      mask Help: Enter the desired 3db rolloff frequency in Hz and the sample time. Initial conditions are sampled automatically.
      mask Display: fprintf('%.2f Hz lowpass',f)
  Add : Sum  Inputs=+-
  Add1 : Sum  Inputs=3  OutDataTypeStr=single
  Add2 : Sum  Inputs=+-  OutDataTypeStr=single
  Add3 : Sum  Inputs=+-  OutDataTypeStr=single
  Add4 : Sum  Inputs=3  OutDataTypeStr=single
  Add5 : Sum  Inputs=+-  OutDataTypeStr=single
  Airspeed Hold [PID] : Subsystem  AncestorBlock=SLUGS_Library/Control Blocks/PID Controller w//Anti-Windup  mask(PID){Tsample=apSampleTime, Ndelay=derivativesConstant, upperSaturationLimit=dtLimit, lowerSaturationLimit=0}
      mask prompts: Tsample "Sample Time"; Ndelay "Integer delays for de/dt"; upperSaturationLimit "Upper Saturation Limit"; lowerSaturationLimit "Lower Saturation Limit"
      mask help: PID controller block with anti-windup and saturation limits. Implemented as a discrete forwardl integration which stops integrating when the output is saturated. Derivative is implemented as a numerical derivative with N integer delays to smooth output.
      mask Display:
      | disp('PID')
      | port_label('input',1,'error')
      | port_label('input',3,'gains')
      | port_label('input',2,'reset')
      | port_label('input',4,'trim')
      | port_label('output',1,'output')
  Constant : Constant  Value=0
  Constant1 : Constant  Value=-3  OutDataTypeStr=single
  Constant2 : Constant  OutDataTypeStr=single
  Constant3 : Constant  Value=2  OutDataTypeStr=single
  Constant4 : Constant  OutDataTypeStr=single
  Elevator  Limit : Saturate  UpperLimit=deLimit  LowerLimit=-deLimit  SampleTime=apSampleTime
  Height Error to Pitch  Command [PI] : Subsystem  AncestorBlock=SLUGS_Library/Control Blocks/PI Controller w//Anti-Windup  mask(PID){Tsample=apSampleTime, Ndelay=derivativesConstant, upperSaturationLimit=pitchCommandLimit, lowerSaturationLimit=-pitchCommandLimit}
      mask prompts: Tsample "Sample Time"; Ndelay "Integer delays for de/dt"; upperSaturationLimit "Upper Saturation Limit"; lowerSaturationLimit "Lower Saturation Limit"
      mask help: PID controller block with anti-windup and saturation limits. Implemented as a discrete forwardl integration which stops integrating when the output is saturated. Derivative is implemented as a numerical derivative with N integer delays to smooth output.
      mask Display:
      | disp('PI')
      | port_label('input',1,'error')
      | port_label('input',3,'gains')
      | port_label('input',2,'reset')
      | port_label('input',4,'trim')
      | port_label('output',1,'output')
  Manual?_1 : InportShadow  Port=12
  Manual?_2 : InportShadow  Port=12
  Pitch To Elevator [PID] : Subsystem  AncestorBlock=SLUGS_Library/Control Blocks/PID Controller w//Anti-Windup  mask(PID){Tsample=apSampleTime, Ndelay=derivativesConstant, upperSaturationLimit=deLimit, lowerSaturationLimit=-deLimit}
      mask prompts: Tsample "Sample Time"; Ndelay "Integer delays for de/dt"; upperSaturationLimit "Upper Saturation Limit"; lowerSaturationLimit "Lower Saturation Limit"
      mask help: PID controller block with anti-windup and saturation limits. Implemented as a discrete forwardl integration which stops integrating when the output is saturated. Derivative is implemented as a numerical derivative with N integer delays to smooth output.
      mask Display:
      | disp('PID')
      | port_label('input',1,'error')
      | port_label('input',3,'gains')
      | port_label('input',2,'reset')
      | port_label('input',4,'trim')
      | port_label('output',1,'output')
  Pitot Control End : SLUGS_Library/Sensor Blocks/Pitot Control End
  Product : Product  Inputs=*/  RndMeth=Zero
  Product1 : Product  RndMeth=Zero
  Product2 : Product  RndMeth=Zero
  Protect NaNs : Subsystem
  Protect NaNs1 : Subsystem
  Protect NaNs2 : Subsystem
  Protect NaNs4 : Subsystem
  Rate Limiter Dynamic with External IC : SLUGS_Library/Singnal Routing & Conditioning/Rate Limiter Dynamic with External IC  rlIC=0
  Selector : Selector  InputPortWidth=3  IndexOptions=Index vector (dialog)  Indices=[1 ]  OutputSizes=1
  Theta_c Limit : Saturate  UpperLimit=pitchCommandLimit  LowerLimit=-pitchCommandLimit  SampleTime=apSampleTime
  Throttle  Limit : Saturate  UpperLimit=dtLimit  LowerLimit=0  SampleTime=apSampleTime
  "[-60 60]" : Saturate  UpperLimit=60  LowerLimit=-60  SampleTime=apSampleTime
  dsPIC_cos : SLUGS_Library/dsPIC_cos
  h_m_1 : InportShadow  Port=6
  theta_m_1 : InportShadow  Port=9
  dE : Outport
  dT : Outport  Port=2
  h_c_in : Outport  Port=3
  U_m : Outport  Port=4
  theta_C : Outport  Port=5
  wires:
  h_c/1 -> Rate Limiter Dynamic with External IC/2
  Constant1/1 -> Rate Limiter Dynamic with External IC/4
  Selector/1 -> Rate Limiter Dynamic with External IC/3
  Constant3/1 -> Rate Limiter Dynamic with External IC/1
  Height Error to Pitch  Command [PI]/1(Output) -> Theta_c Limit/1
  Rate Limiter Dynamic with External IC/1 -> Add2/1, h_c_in/1
  Theta_c Limit/1 -> Add3/1, theta_C/1
  Add3/1 -> Protect NaNs2/1(In1)
  th2dE PID Gains/1 -> Pitch To Elevator [PID]/3(PIDGains)
  he2th PI Gains/1 -> Height Error to Pitch  Command [PI]/3(PIDGains)
  h_m_1/1 -> Pitot Control End/2
  dyn P/1 -> Pitot Control End/1
  Elevator  Limit/1 -> dE/1
  dE_trim/1 -> Add4/2, Pitch To Elevator [PID]/4(Trim)
  Pitch To Elevator [PID]/1(Output) -> Add4/1
  Add4/1 -> Elevator  Limit/1
  Manual?_2/1 -> Pitch To Elevator [PID]/2(Reset)
  Manual?_1/1 -> Height Error to Pitch  Command [PI]/2(Reset)
  Manual?/1 -> Airspeed Hold [PID]/2(Reset)
  theta_m/1 -> Add3/2
  h_m/1 -> Add2/2
  Add2/1 -> Protect NaNs1/1(In1)
  Throttle  Limit/1 -> dT/1
  Add1/1 -> Throttle  Limit/1
  dT_trim/1 -> Add1/2, Airspeed Hold [PID]/4(Trim)
  Airspeed Hold [PID]/1(Output) -> Add1/1
  Add/1 -> Protect NaNs/1(In1)
  U_c/1 -> Add/1
  Pitot Control End/1 -> Add/2, U_m/1
  phi_m/1 -> Protect NaNs4/1(In1)
  Constant2/1 -> Add5/2
  dsPIC_cos/1 -> Product/2
  Constant4/1 -> Product/1
  Product/1 -> Add5/1
  0.5 sec  tau for Turns/1(Out1) -> "[-60 60]"/1
  "[-60 60]"/1 -> dsPIC_cos/1
  Add5/1 -> Product1/2
  Roll to Height FF/1 -> Product1/1
  Product1/1 -> Add4/3
  theta_m_1/1 -> Product2/2
  Product2/1 -> Add1/3
  dt FF Gain/1 -> Product2/1
  U_hold PID  Gains/1 -> Airspeed Hold [PID]/3(PIDGains)
  Constant/1 -> Height Error to Pitch  Command [PI]/4(Trim)
  Protect NaNs/1(Out1) -> Airspeed Hold [PID]/1(Error)
  Protect NaNs1/1(Out1) -> Height Error to Pitch  Command [PI]/1(Error)
  Protect NaNs2/1(Out1) -> Pitch To Elevator [PID]/1(Error)
  Protect NaNs4/1(Out1) -> 0.5 sec  tau for Turns/1(In1)
  GS Location/1 -> Selector/1

== system SLUGS_Library/Control Blocks/psi_dot_c Select logic ==
  psi_dot_ad : Inport
  L1OnOff : Inport  Port=2
  psi_dot_c_noNav : Inport  Port=3
  IsPassThrough : Inport  Port=4
  nav_phi_c : Inport  Port=5
  U_m : Inport  Port=6
  Bank to Psi Dot : Subsystem  AncestorBlock=SLUGS_Library/Navigation/Bank to Psi Dot
  Switch : Switch  Criteria=u2 > Threshold  Threshold=0.3
  Switch1 : Switch  Criteria=u2 > Threshold  Threshold=0.3  InputSameDT=on
  psi_dot_c : Outport
  psi_dot_c_4_L1 : Outport  Port=2
  wires:
  Bank to Psi Dot/1(psi_dot_c) -> Switch1/3
  Switch1/1 -> Switch/3, psi_dot_c_4_L1/1
  psi_dot_ad/1 -> Switch/1
  L1OnOff/1 -> Switch/2
  Switch/1 -> psi_dot_c/1
  psi_dot_c_noNav/1 -> Switch1/1
  IsPassThrough/1 -> Switch1/2
  nav_phi_c/1 -> Bank to Psi Dot/1(phi_c)
  U_m/1 -> Bank to Psi Dot/2(U_m)

== system SLUGS_Library/InnerLoop/Lateral Channel ==
  r_m : Inport
  Manual? : Inport  Port=2
  Yaw Damp  PID Gains : Inport  Port=3
  dR Trim : Inport  Port=4
  psi_dot_c : Inport  Port=5
  U_m : Inport  Port=6
  phi_m : Inport  Port=7
  Roll PID Gains : Inport  Port=8
  dA Trim : Inport  Port=9
  wpFly : Inport  Port=10  SampleTime=apSampleTime
  nav_phi_c : Inport  Port=11
  Add : Sum  OutDataTypeStr=single
  Add1 : Sum  Inputs=-+  OutDataTypeStr=single
  Add3 : Sum  OutDataTypeStr=single
  Aileron Limit : Saturate  UpperLimit=daLimit  LowerLimit=-daLimit  SampleTime=apSampleTime
  Bank  Limit Command : Saturate  UpperLimit=bankCommandLimit  LowerLimit=-bankCommandLimit  SampleTime=apSampleTime
  Bank to Psi Dot : SLUGS_Library/Navigation/Bank to Psi Dot
  Constant : Constant  Value=0  OutDataTypeStr=single
  Constant1 : Constant  Value=0  OutDataTypeStr=single
  Data Type Conversion3 : DataTypeConversion  OutDataTypeStr=single
  High Pass (Washout) Filter : SLUGS_Library/Singnal Routing & Conditioning/Filter  Zeros=[0]  Poles=[-1/5]  Gain=1  AbsTol=auto  SampleTime=apSampleTime  method=tustin  Wc=1
  Manual?1 : InportShadow  Port=2
  Neg Feedback : Gain  Gain=-1  OutDataTypeStr=float('double')
  Roll Control : SLUGS_Library/Control Blocks/PID Controller  TSample=apSampleTime  NDelay=derivativesConstant  upperLimit=rollControlLimit  lowerLimit=-rollControlLimit
  Rudder Limit : Saturate  UpperLimit=apSampleTime  LowerLimit=-drLimit  SampleTime=apSampleTime
  Switch : Switch  Criteria=u2 > Threshold  Threshold=0.3
  Switch1 : Switch  Criteria=u2 > Threshold  Threshold=0.3  InputSameDT=on
  Yaw Damper : SLUGS_Library/Control Blocks/PID Controller  TSample=apSampleTime  NDelay=derivativesConstant  upperLimit=yawDamperLimit  lowerLimit=-yawDamperLimit
  "nav_phi_c  " : InportShadow  Port=11
  psi_dot to Bank : SLUGS_Library/Navigation/psi_dot to Bank
  psi_dot_c1 : InportShadow  Port=5
  "wpFly " : InportShadow  Port=10  SampleTime=apSampleTime
  dA : Outport
  dR : Outport  Port=2
  phi_c : Outport  Port=3
  "psi_dot_c " : Outport  Port=4
  wires:
  High Pass (Washout) Filter/1 -> Data Type Conversion3/1
  Neg Feedback/1 -> High Pass (Washout) Filter/1
  r_m/1 -> Neg Feedback/1
  Rudder Limit/1 -> dR/1
  Constant/1 -> Yaw Damper/3
  Manual?/1 -> Yaw Damper/2
  Yaw Damp  PID Gains/1 -> Yaw Damper/4
  Add/1 -> Rudder Limit/1
  Yaw Damper/1 -> Add/1
  dR Trim/1 -> Add/2
  psi_dot_c/1 -> psi_dot to Bank/1
  U_m/1 -> Bank to Psi Dot/2, psi_dot to Bank/2
  Manual?1/1 -> Roll Control/2
  Constant1/1 -> Roll Control/3
  Roll PID Gains/1 -> Roll Control/4
  Add3/1 -> Aileron Limit/1
  Roll Control/1 -> Add3/1
  dA Trim/1 -> Add3/2
  Aileron Limit/1 -> dA/1
  Add1/1 -> Roll Control/1
  phi_m/1 -> Add1/1
  Switch/1 -> Bank  Limit Command/1
  nav_phi_c/1 -> Switch/1
  wpFly/1 -> Switch/2
  psi_dot to Bank/1 -> Switch/3
  Bank  Limit Command/1 -> Add1/2, phi_c/1
  "wpFly "/1 -> Switch1/2
  Switch1/1 -> "psi_dot_c "/1
  "nav_phi_c  "/1 -> Bank to Psi Dot/1
  Bank to Psi Dot/1 -> Switch1/1
  psi_dot_c1/1 -> Switch1/3
  Data Type Conversion3/1 -> Yaw Damper/1
